simulink model "QUAD_With_MPC_Final"  (R2015a)
settings: Solver=ode45  StartTime=0.0  StopTime=120  RelTol=1e-3
libraries: simulink x6, commnoisgen2 x5, mpclib x1
settings Model: SimulationMode=accelerator  Creator=Oussama  LastModifiedBy=Oussama

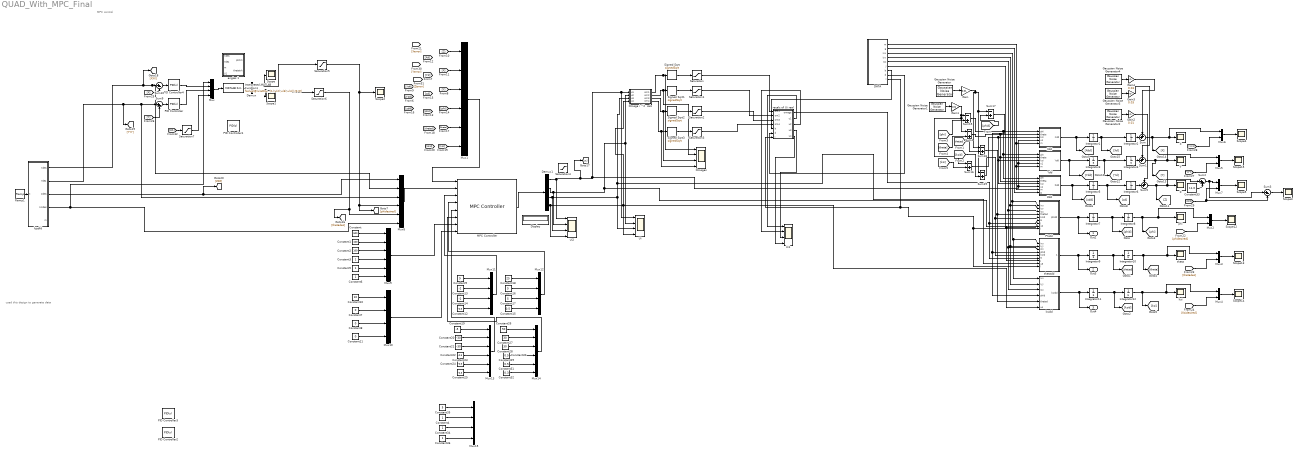
== system QUAD_With_MPC_Final ==
  note: MPC control
  note: used this design to generate data
  Constant : Constant  Value=500
  Constant1 : Constant  Value=100
  Constant10 : Constant  Value=10
  Constant11 : Constant  Value=0
  Constant12 : Constant  Value=-0.5
  Constant13 : Constant  Value=-2
  Constant14 : Constant  Value=-2
  Constant15 : Constant  Value=0.5
  Constant16 : Constant  Value=5
  Constant17 : Constant  Value=5
  Constant18 : Constant  Value=25
  Constant19 : Constant  Value=-5
  Constant2 : Constant  Value=100
  Constant20 : Constant  Value=-30
  Constant21 : Constant  Value=-30
  Constant{3..6,22,29,34,36} (8 alike) : Constant
  Constant23 : Constant  Value=-0.5
  Constant24 : Constant  Value=-0.5
  Constant25 : Constant  Value=-0.3
  Constant26 : Constant  Value=50
  Constant27 : Constant  Value=30
  Constant28 : Constant  Value=30
  Constant30 : Constant  Value=0.5
  Constant31 : Constant  Value=0.5
  Constant32 : Constant  Value=0.3
  Constant33 : Constant  Value=11.0
  Constant35 : Constant  Value=5
  Constant7 : Constant  Value=0
  Constant8 : Constant  Value=0
  Constant9 : Constant  Value=9
  DATA : MATLAB Function  TreatAsAtomicUnit=on
  Demux : Demux  Outputs=2
  Demux1 : Demux
  Display : Display
  Gain : Gain  Gain=0.01
  Gain1 : Gain  Gain=0.01
  Gain2 : Gain  Gain=0.01
  Gain3 : Gain  Gain=0.03
  Gain4 : Gain  Gain=0.03
  Gaussian Noise Generator : commnoisgen2/Gaussian Noise Generator  m=0  d=1  s=41  Ts=0.07  frameBased=off  sampPerFrame=1  orient=off  outDataType=double
  Gaussian Noise Generator1 : commnoisgen2/Gaussian Noise Generator  m=0  d=1  s=41  Ts=0.07  frameBased=off  sampPerFrame=1  orient=off  outDataType=double
  Gaussian Noise Generator2 : commnoisgen2/Gaussian Noise Generator  m=0.3  d=1  s=41  Ts=0.5  frameBased=off  sampPerFrame=1  orient=off  outDataType=double
  Gaussian Noise Generator3 : commnoisgen2/Gaussian Noise Generator  m=0.3  d=1  s=41  Ts=1.2  frameBased=off  sampPerFrame=1  orient=off  outDataType=double
  Gaussian Noise Generator4 : commnoisgen2/Gaussian Noise Generator  m=0.3  d=1  s=41  Ts=1  frameBased=off  sampPerFrame=1  orient=off  outDataType=double
  Integrator{1..12} (12 alike) : Integrator
  Interpreted MATLAB Function1 : MATLABFcn  MATLABFcn=fsolve(@(x)attitudes3(x,u(1),u(2),u(3),u(4)),[0,0])  OutputDimensions=2
  MPC Controller : mpclib/MPC Controller  SCDEnableBlockLinearizationSpecification=on  mpcobj=MPC2  is_multiple=0  enable_value=0  n_mv=4  n_mo=6  n_md=0  n_ts=0.02  is_designfromscratch=0  return_u0=off  ref_from_ws=off  ref_signal_name=[]  ref_preview=off  md_from_ws=off  md_signal_name=[]  md_preview=off  from_project=off  project_file=MPCtask.mat  md_inport=off  mv_inport=off  cost_outport=off  return_sequence=off  return_qpstatus=off  return_state=off  state_inport=off  lims_inport=on  ywt_inport=on  uwt_inport=off  duwt_inport=off  rhoeps_inport=off  uref_inport=on  BlockDataType=double  SampleTimeInherited=off  switch_inport=off
  Mux{,10..12,15} (5 alike) : Mux
  Mux{1,8..9,13..14} (5 alike) : Mux  Inputs=6
  Mux{2..7} (6 alike) : Mux  Inputs=2
  Omega i ^2  calc : MATLAB Function  TreatAsAtomicUnit=on
  Omegas : Scope  NumInputPorts=4
      settings: YMin=-5~-5~-5~-5  YMax=5~5~5~5  SaveName=ScopeData3
  PID Controller : simulink/Continuous/PID Controller  Controller=PID  TimeDomain=Continuous-time  SampleTime=-1  IntegratorMethod=Forward Euler  FilterMethod=Forward Euler  Form=Parallel  UseFilter=on  ControllerParametersSource=internal  P=0.7  I=0.4  D=1.8  N=100  InitialConditionSource=internal  InitialConditionForIntegrator=0  InitialConditionForFilter=0  ExternalReset=none  LimitOutput=off  UpperSaturationLimit=inf  LowerSaturationLimit=-inf  LinearizeAsGain=on  AntiWindupMode=none  Kb=1  TrackingMode=off  Kt=1  PParamMin=[]  PParamMax=[]  IParamMin=[]  IParamMax=[]  DParamMin=[]  DParamMax=[]  NParamMin=[]  NParamMax=[]  KbParamMin=[]  KbParamMax=[]  KtParamMin=[]  KtParamMax=[]  POutMin=[]  POutMax=[]  IOutMin=[]  IOutMax=[]  DOutMin=[]  DOutMax=[]  NOutMin=[]  NOutMax=[]  KbOutMin=[]  KbOutMax=[]  KtOutMin=[]  KtOutMax=[]  IntegratorOutMin=[]  IntegratorOutMax=[]  FilterOutMin=[]  FilterOutMax=[]  SumOutMin=[]  SumOutMax=[]  SumI1OutMin=[]  SumI1OutMax=[]  SumI2OutMin=[]  SumI2OutMax=[]  SumI3OutMin=[]  SumI3OutMax=[]  SumDOutMin=[]  SumDOutMax=[]  SaturationOutMin=[]  SaturationOutMax=[]  IntegratorContinuousStateAttributes=''  IntegratorStateMustResolveToSignalObject=off  IntegratorRTWStateStorageClass=Auto  FilterContinuousStateAttributes=''  FilterStateMustResolveToSignalObject=off  FilterRTWStateStorageClass=Auto  DifferentiatorICPrevScaledInput=0  DifferentiatorOutMin=[]  DifferentiatorOutMax=[]
  PID Controller1 : simulink/Continuous/PID Controller  Controller=PID  TimeDomain=Continuous-time  SampleTime=-1  IntegratorMethod=Forward Euler  FilterMethod=Forward Euler  Form=Parallel  UseFilter=on  ControllerParametersSource=internal  P=1  I=0.7  D=2.9  N=100  InitialConditionSource=internal  InitialConditionForIntegrator=0  InitialConditionForFilter=0  ExternalReset=none  LimitOutput=off  UpperSaturationLimit=inf  LowerSaturationLimit=-inf  LinearizeAsGain=on  AntiWindupMode=none  Kb=1  TrackingMode=off  Kt=1  PParamMin=[]  PParamMax=[]  IParamMin=[]  IParamMax=[]  DParamMin=[]  DParamMax=[]  NParamMin=[]  NParamMax=[]  KbParamMin=[]  KbParamMax=[]  KtParamMin=[]  KtParamMax=[]  POutMin=[]  POutMax=[]  IOutMin=[]  IOutMax=[]  DOutMin=[]  DOutMax=[]  NOutMin=[]  NOutMax=[]  KbOutMin=[]  KbOutMax=[]  KtOutMin=[]  KtOutMax=[]  IntegratorOutMin=[]  IntegratorOutMax=[]  FilterOutMin=[]  FilterOutMax=[]  SumOutMin=[]  SumOutMax=[]  SumI1OutMin=[]  SumI1OutMax=[]  SumI2OutMin=[]  SumI2OutMax=[]  SumI3OutMin=[]  SumI3OutMax=[]  SumDOutMin=[]  SumDOutMax=[]  SaturationOutMin=[]  SaturationOutMax=[]  IntegratorContinuousStateAttributes=''  IntegratorStateMustResolveToSignalObject=off  IntegratorRTWStateStorageClass=Auto  FilterContinuousStateAttributes=''  FilterStateMustResolveToSignalObject=off  FilterRTWStateStorageClass=Auto  DifferentiatorICPrevScaledInput=0  DifferentiatorOutMin=[]  DifferentiatorOutMax=[]
  PID Controller2 : simulink/Continuous/PID Controller  Controller=PID  TimeDomain=Continuous-time  SampleTime=-1  IntegratorMethod=Forward Euler  FilterMethod=Forward Euler  Form=Parallel  UseFilter=on  ControllerParametersSource=internal  P=0.5  I=0.1  D=0.25  N=100  InitialConditionSource=internal  InitialConditionForIntegrator=0  InitialConditionForFilter=0  ExternalReset=none  LimitOutput=off  UpperSaturationLimit=inf  LowerSaturationLimit=-inf  LinearizeAsGain=on  AntiWindupMode=none  Kb=1  TrackingMode=off  Kt=1  PParamMin=[]  PParamMax=[]  IParamMin=[]  IParamMax=[]  DParamMin=[]  DParamMax=[]  NParamMin=[]  NParamMax=[]  KbParamMin=[]  KbParamMax=[]  KtParamMin=[]  KtParamMax=[]  POutMin=[]  POutMax=[]  IOutMin=[]  IOutMax=[]  DOutMin=[]  DOutMax=[]  NOutMin=[]  NOutMax=[]  KbOutMin=[]  KbOutMax=[]  KtOutMin=[]  KtOutMax=[]  IntegratorOutMin=[]  IntegratorOutMax=[]  FilterOutMin=[]  FilterOutMax=[]  SumOutMin=[]  SumOutMax=[]  SumI1OutMin=[]  SumI1OutMax=[]  SumI2OutMin=[]  SumI2OutMax=[]  SumI3OutMin=[]  SumI3OutMax=[]  SumDOutMin=[]  SumDOutMax=[]  SaturationOutMin=[]  SaturationOutMax=[]  IntegratorContinuousStateAttributes=''  IntegratorStateMustResolveToSignalObject=off  IntegratorRTWStateStorageClass=Auto  FilterContinuousStateAttributes=''  FilterStateMustResolveToSignalObject=off  FilterRTWStateStorageClass=Auto  DifferentiatorICPrevScaledInput=0  DifferentiatorOutMin=[]  DifferentiatorOutMax=[]
  PID Controller3 : simulink/Continuous/PID Controller  Controller=PID  TimeDomain=Continuous-time  SampleTime=-1  IntegratorMethod=Forward Euler  FilterMethod=Forward Euler  Form=Parallel  UseFilter=on  ControllerParametersSource=internal  P=0.5  I=0.1  D=0.3  N=100  InitialConditionSource=internal  InitialConditionForIntegrator=0  InitialConditionForFilter=0  ExternalReset=none  LimitOutput=off  UpperSaturationLimit=inf  LowerSaturationLimit=-inf  LinearizeAsGain=on  AntiWindupMode=none  Kb=1  TrackingMode=off  Kt=1  PParamMin=[]  PParamMax=[]  IParamMin=[]  IParamMax=[]  DParamMin=[]  DParamMax=[]  NParamMin=[]  NParamMax=[]  KbParamMin=[]  KbParamMax=[]  KtParamMin=[]  KtParamMax=[]  POutMin=[]  POutMax=[]  IOutMin=[]  IOutMax=[]  DOutMin=[]  DOutMax=[]  NOutMin=[]  NOutMax=[]  KbOutMin=[]  KbOutMax=[]  KtOutMin=[]  KtOutMax=[]  IntegratorOutMin=[]  IntegratorOutMax=[]  FilterOutMin=[]  FilterOutMax=[]  SumOutMin=[]  SumOutMax=[]  SumI1OutMin=[]  SumI1OutMax=[]  SumI2OutMin=[]  SumI2OutMax=[]  SumI3OutMin=[]  SumI3OutMax=[]  SumDOutMin=[]  SumDOutMax=[]  SaturationOutMin=[]  SaturationOutMax=[]  IntegratorContinuousStateAttributes=''  IntegratorStateMustResolveToSignalObject=off  IntegratorRTWStateStorageClass=Auto  FilterContinuousStateAttributes=''  FilterStateMustResolveToSignalObject=off  FilterRTWStateStorageClass=Auto  DifferentiatorICPrevScaledInput=0  DifferentiatorOutMin=[]  DifferentiatorOutMax=[]
  PID Controller4 : simulink/Continuous/PID Controller  Controller=PID  TimeDomain=Continuous-time  SampleTime=-1  IntegratorMethod=Forward Euler  FilterMethod=Forward Euler  Form=Parallel  UseFilter=on  ControllerParametersSource=internal  P=0.7  I=0.4  D=1.8  N=100  InitialConditionSource=internal  InitialConditionForIntegrator=0  InitialConditionForFilter=0  ExternalReset=none  LimitOutput=off  UpperSaturationLimit=inf  LowerSaturationLimit=-inf  LinearizeAsGain=on  AntiWindupMode=none  Kb=1  TrackingMode=off  Kt=1  PParamMin=[]  PParamMax=[]  IParamMin=[]  IParamMax=[]  DParamMin=[]  DParamMax=[]  NParamMin=[]  NParamMax=[]  KbParamMin=[]  KbParamMax=[]  KtParamMin=[]  KtParamMax=[]  POutMin=[]  POutMax=[]  IOutMin=[]  IOutMax=[]  DOutMin=[]  DOutMax=[]  NOutMin=[]  NOutMax=[]  KbOutMin=[]  KbOutMax=[]  KtOutMin=[]  KtOutMax=[]  IntegratorOutMin=[]  IntegratorOutMax=[]  FilterOutMin=[]  FilterOutMax=[]  SumOutMin=[]  SumOutMax=[]  SumI1OutMin=[]  SumI1OutMax=[]  SumI2OutMin=[]  SumI2OutMax=[]  SumI3OutMin=[]  SumI3OutMax=[]  SumDOutMin=[]  SumDOutMax=[]  SaturationOutMin=[]  SaturationOutMax=[]  IntegratorContinuousStateAttributes=''  IntegratorStateMustResolveToSignalObject=off  IntegratorRTWStateStorageClass=Auto  FilterContinuousStateAttributes=''  FilterStateMustResolveToSignalObject=off  FilterRTWStateStorageClass=Auto  DifferentiatorICPrevScaledInput=0  DifferentiatorOutMin=[]  DifferentiatorOutMax=[]
  Phidd : MATLAB Function  TreatAsAtomicUnit=on
  Ramp1 : simulink/Sources/Ramp  slope=1  start=0  X0=0
  Saturation{,1..3} (4 alike) : Saturate  UpperLimit=5000  LowerLimit=0
  Saturation4 : Saturate  UpperLimit=50  LowerLimit=5
  Saturation5 : Saturate  UpperLimit=0.4  LowerLimit=-0.4
  Saturation6 : Saturate
  Saturation7 : Saturate  UpperLimit=50  LowerLimit=0.5
  Scope{,1..5,12..15} (10 alike) : Scope
      Scope settings: TimeRange=10  YMin=-0.504  YMax=-0.491
      Scope1 settings: YMin=1.49226  YMax=1.64934
      Scope12 settings: YMin=-0.00625  YMax=-0.00425  SaveName=phi_ang
      Scope13 settings: YMin=-0.07  YMax=0.05  SaveName=theta_ang
      Scope14 settings: YMin=0  YMax=7e-13  SaveName=psi_ang
      Scope15 settings: YMin=-9.78  YMax=-9.65  SaveName=ydata
      Scope2 settings: YMin=1.49226  YMax=1.64934  SaveName=ScopeData8
      Scope3 settings: YMin=-12.016  YMax=-12.006  SaveName=zdata1
      Scope4 settings: TimeRange=44.14385330578512  YMin=0  YMax=13  SaveName=xdata
      Scope5 settings: YMin=7.95  YMax=8.5  SaveName=zdata
  Signed Sqrt{,1..3} (4 alike) : Sqrt  Operator=signedSqrt  SaturateOnIntegerOverflow=on
  Sum : Sum  Inputs=++|
  Sum1 : Sum  Inputs=++|
  Sum10 : Sum  Inputs=|+-
  Sum{4,15..19} (6 alike) : Sum  Inputs=-+
  Sum2 : Sum  Inputs=|++
  Sum3 : Sum  Inputs=|+-
  Sum5 : Sum  Inputs=++|
  Sum9 : Sum  Inputs=|+-
  Ui : Scope  NumInputPorts=4
      settings: YMin=-5~-5~-5~-5  YMax=5~5~5~5  SaveName=ScopeData15
  Ui1 : Scope  NumInputPorts=4
      settings: YMin=-5~-5~-5~-5  YMax=5~5~5~5  SaveName=ScopeData4
  Ui2 : Scope  NumInputPorts=4
      settings: YMin=-5~-5~-5~-5  YMax=5~5~5~5  SaveName=ScopeData7
  X : Scope
      settings: YMin=3.81  YMax=3.95  SaveName=ScopeData6
  Xdd : MATLAB Function  TreatAsAtomicUnit=on
  Y : Scope
      settings: YMin=-0.01095  YMax=-0.0103  SaveName=ScopeData5
  Ydd : MATLAB Function  TreatAsAtomicUnit=on
  "Z " : Scope
      settings: YMin=7.615  YMax=7.6215  SaveName=ScopeData2
  Zdd : MATLAB Function  TreatAsAtomicUnit=on
  angles 1 : MATLAB Function  TreatAsAtomicUnit=on
  "hjsdfd " : MATLAB Function  TreatAsAtomicUnit=on
  ksi : Scope
      settings: SaveName=ksiangle
  ksidd : MATLAB Function  TreatAsAtomicUnit=on
  phi : Scope
      settings: SaveName=phiangle
  recalc of Ui real : MATLAB Function  TreatAsAtomicUnit=on
  theta : Scope
      settings: SaveName=thetaangle
  thetadd : MATLAB Function  TreatAsAtomicUnit=on
  Out2 : Outport
  Out3 : Outport  Port=2
  Out4 : Outport  Port=3
  wires:
  Saturation/1 -> recalc of Ui real/1(om1)
  Saturation1/1 -> recalc of Ui real/2(om2)
  Saturation2/1 -> recalc of Ui real/3(om3)
  Signed Sqrt/1 -> Saturation/1
  Signed Sqrt1/1 -> Saturation1/1
  Signed Sqrt2/1 -> Saturation2/1
  Signed Sqrt3/1 -> Saturation3/1
  Xdd/1(Xdd) -> [Xdd], Integrator1/1
  Ydd/1(Ydd) -> [Ydd], Integrator3/1
  Zdd/1(Zdd) -> [zdd], Integrator5/1
  Phidd/1(phidd) -> Out2/1, Integrator7/1
  Integrator7/1 -> [phid], Integrator8/1
  thetadd/1(thetadd) -> Out3/1, Integrator9/1
  Integrator9/1 -> [thetad], Integrator10/1
  ksidd/1(ksidd) -> Out4/1, Integrator11/1
  Integrator11/1 -> [ksid], Integrator12/1
  Integrator8/1 -> Mux2/1, phi/1, [phi]
  DATA/1(m) -> Zdd/5(m), Ydd/5(m), Xdd/5(m)
  DATA/2(g) -> Zdd/6(g)
  DATA/3(Ixx) -> ksidd/1(Ixx), thetadd/1(Ixx), Phidd/1(Ixx)
  DATA/4(Iyy) -> Phidd/2(Iyy), ksidd/2(Iyy), thetadd/2(Iyy)
  DATA/5(Izz) -> thetadd/3(Izz), ksidd/3(Izz), Phidd/3(Izz)
  DATA/6(J) -> thetadd/7(J), Phidd/7(J)
  Sum15/1 -> Zdd/1(phi), Ydd/1(phi), Xdd/1(phi)
  Sum4/1 -> Zdd/2(theta), Ydd/2(theta), Xdd/2(theta)
  Sum16/1 -> Ydd/3(ksi), Zdd/3(ksi), Xdd/3(ksi)
  Sum18/1 -> Phidd/4(thetad), ksidd/5(thetad)
  Sum19/1 -> Phidd/5(ksid), thetadd/5(ksid)
  Sum17/1 -> ksidd/4(phid), thetadd/4(phid)
  recalc of Ui real/1(omega) -> thetadd/6(omega), Phidd/6(omega)
  DATA/7(b) -> recalc of Ui real/5(b)
  DATA/8(d) -> recalc of Ui real/6(d)
  Demux1/4 -> Ui2/4, Omega i ^2  calc/4(u4), Ui/4, ksidd/6(u4)
  Demux1/3 -> Ui2/3, Omega i ^2  calc/3(u3), thetadd/8(u3), Ui/3
  Demux1/2 -> Ui2/2, Phidd/8(u2), Omega i ^2  calc/2(u2), Ui/2
  Omega i ^2  calc/1(om1) -> Omegas/1, Signed Sqrt/1
  Omega i ^2  calc/2(om2) -> Omegas/2, Signed Sqrt1/1
  Omega i ^2  calc/3(om3) -> Omegas/3, Signed Sqrt2/1
  Omega i ^2  calc/4(om4) -> Omegas/4, Signed Sqrt3/1
  Gain1/1 -> Sum16/1, Sum4/1, Sum15/1
  [phi] -> Sum15/2
  [theta] -> Sum4/2
  [ksi] -> Sum16/2
  Gain/1 -> Sum19/1, Sum17/1, Sum18/1
  [phid] -> Sum17/2
  [thetad] -> Sum18/2
  [ksid] -> Sum19/2
  Integrator5/1 -> [zd], Integrator6/1
  Integrator3/1 -> [Yd], Integrator4/1
  Integrator1/1 -> [Xd], Integrator2/1
  DATA/9(l) -> Phidd/9(l), thetadd/9(l), recalc of Ui real/7(l)
  [phidesired] -> Mux2/2
  Mux2/1 -> Scope12/1
  Integrator10/1 -> [theta], Mux3/1, theta/1
  [thetades] -> Mux3/2
  Mux3/1 -> Scope13/1
  Integrator12/1 -> [ksi], Mux4/1, ksi/1
  [Ksidesired] -> Mux4/2
  Mux4/1 -> Scope14/1
  "hjsdfd "/1(Xdes) -> Mux8/2, Sum10/1, [XXX]
  [X] -> Sum10/2
  "hjsdfd "/2(Ydes) -> Mux8/3, Sum9/1, [YYY]
  [Y] -> Sum9/2
  Mux5/1 -> Scope15/1
  Sum/1 -> [X], Mux6/1, X/1
  [XXX] -> Mux6/2
  [ZZZ] -> Sum3/2, Mux7/2
  [X] -> Mux1/2
  [Y] -> Mux1/3
  [phi] -> Mux1/4
  [theta] -> Mux1/5
  [ksi] -> Mux1/6
  Mux1/1 -> MPC Controller/1
  Mux8/1 -> MPC Controller/2
  MPC Controller/1 -> Demux1/1
  Mux/1 -> Interpreted MATLAB Function1/1
  Demux/1 -> Scope/1, Saturation5/1
  Demux/2 -> Saturation6/1, Scope1/1
  Interpreted MATLAB Function1/1 -> Demux/1
  "hjsdfd "/4(ksides) -> Mux/1, Mux8/6
  Sum10/1 -> PID Controller4/1
  Sum9/1 -> PID Controller/1
  Saturation6/1 -> Mux8/5, [thetades]
  Saturation5/1 -> Scope2/1, Mux8/4, [phidesired]
  Sum1/1 -> [Y], Mux5/1, Y/1
  [YYY] -> Mux5/2
  Sum5/1 -> [Z], Sum2/1, "Z "/1
  Mux7/1 -> Scope5/1
  Saturation3/1 -> recalc of Ui real/4(om4)
  Mux9/1 -> MPC Controller/7
  Constant/1 -> Mux9/1
  Constant1/1 -> Mux9/2
  Constant2/1 -> Mux9/3
  Constant3/1 -> Mux9/4
  Constant5/1 -> Mux9/5
  Constant6/1 -> Mux9/6
  Mux10/1 -> MPC Controller/8
  Constant7/1 -> Mux10/2
  Constant8/1 -> Mux10/3
  Constant10/1 -> Mux10/1
  Constant11/1 -> Mux10/4
  Mux11/1 -> MPC Controller/3
  Constant13/1 -> Mux11/2
  Constant14/1 -> Mux11/3
  Constant9/1 -> Mux11/1
  Constant12/1 -> Mux11/4
  Constant16/1 -> Mux12/2
  Constant17/1 -> Mux12/3
  Constant18/1 -> Mux12/1
  Constant15/1 -> Mux12/4
  Mux12/1 -> MPC Controller/4
  Mux13/1 -> MPC Controller/5
  Constant19/1 -> Mux13/1
  Constant20/1 -> Mux13/2
  Constant21/1 -> Mux13/3
  Constant22/1 -> Mux13/4
  Constant24/1 -> Mux13/5
  Constant25/1 -> Mux13/6
  Mux14/1 -> MPC Controller/6
  Constant26/1 -> Mux14/1
  Constant27/1 -> Mux14/2
  Constant28/1 -> Mux14/3
  Constant29/1 -> Mux14/4
  Constant31/1 -> Mux14/5
  Constant32/1 -> Mux14/6
  recalc of Ui real/2(u1) -> Ui1/1
  recalc of Ui real/3(u2) -> Ui1/2
  recalc of Ui real/4(u3) -> Ui1/3
  recalc of Ui real/5(u4) -> Ui1/4
  PID Controller/1 -> Mux/3
  PID Controller4/1 -> Mux/2
  "hjsdfd "/3(Zdes) -> [ZZZ], Mux8/1
  Sum2/1 -> Sum3/1, Mux7/1
  Constant33/1 -> Sum2/2
  Sum3/1 -> Scope3/1
  [Z] -> Mux1/1
  Constant4/1 -> Mux15/2
  Constant34/1 -> Mux15/3
  Constant35/1 -> Mux15/1
  Constant36/1 -> Mux15/4
  [U1] -> Saturation7/1
  Saturation7/1 -> Mux/4
  Mux6/1 -> Scope4/1
  Ramp1/1 -> "hjsdfd "/1(t)
  Gaussian Noise Generator2/1 -> Gain2/1
  Gain2/1 -> Sum5/1
  Gaussian Noise Generator3/1 -> Gain3/1
  Gain3/1 -> Sum1/1
  Gaussian Noise Generator4/1 -> Gain4/1
  Gain4/1 -> Sum/1
  Gaussian Noise Generator/1 -> Gain/1
  Gaussian Noise Generator1/1 -> Gain1/1
  Integrator2/1 -> Sum/2
  Integrator4/1 -> Sum1/2
  Integrator6/1 -> Sum5/2
  Demux1/1 -> [U1], Zdd/4(u1), Ydd/4(u1), Xdd/4(u1), Omega i ^2  calc/1(u1), Ui/1, Ui2/1

== matlab function QUAD_With_MPC_Final/Ydd ==
  data: phi input; Ydd output; theta input; ksi input; u1 input; m input
function Ydd = fcn(phi,theta, ksi,u1,m)
m=1;

Ydd=(-cos(ksi)*sin(phi)+sin(ksi)*sin(theta)*cos(phi))*u1/m;

== matlab function QUAD_With_MPC_Final/Zdd ==
  data: phi input; Zdd output; theta input; ksi input; u1 input; m input; g input
function Zdd = fcn(phi,theta, ksi,u1,m,g)
m=1;
g=9.81;

Zdd=-g+(cos(theta)*cos(phi))*u1/m;

== matlab function QUAD_With_MPC_Final/DATA ==
  data: m output; g output; Ixx output; Iyy output; Izz output; J output; b output; d output; l output
function [m,g,Ixx,Iyy,Izz,J,b,d,l] = fcn
m=1;
g=9.81;

Ixx=1*0.008;
Iyy=1*0.008;
Izz=1*0.015;
b=0.0001;
d=0.000001;
l=0.25;
J=0.0001;

== matlab function QUAD_With_MPC_Final/Phidd ==
  data: Ixx input; Iyy input; phidd output; Izz input; thetad input; ksid input; omega input; J input; u2 input; l input
function phidd = fcn(Ixx,Iyy,Izz,thetad, ksid,omega,J,u2,l)


phidd=1/Ixx*((Iyy-Izz)*thetad*ksid-J*thetad*omega+l*u2);

== matlab function QUAD_With_MPC_Final/thetadd ==
  data: Ixx input; Iyy input; thetadd output; Izz input; phid input; ksid input; omega input; J input; u3 input; l input
function thetadd = fcn(Ixx,Iyy,Izz,phid, ksid,omega,J,u3,l)


thetadd=1/Iyy*((Izz-Ixx)*phid*ksid+J*phid*omega+l*u3);

== matlab function QUAD_With_MPC_Final/ksidd ==
  data: Ixx input; Iyy input; ksidd output; Izz input; phid input; thetad input; u4 input
function ksidd = fcn(Ixx,Iyy,Izz,phid, thetad,u4)


ksidd=1/Izz*((Ixx-Iyy)*phid*thetad+u4);

== matlab function QUAD_With_MPC_Final/Omega i ^2  calc ==
  data: u1 input; om1 output; u2 input; u3 input; u4 input; om2 output; om3 output; om4 output
function [om1,om2,om3,om4] = fcn(u1,u2,u3,u4)
%#codegen
b=0.0001;
d=0.000001;
l=0.25;
A=[ 1/(4*b),0, -1/(2*b*l), -1/(4*d);1/(4*b), -1/(2*b*l),0,  1/(4*d); 1/(4*b),  0,  1/(2*b*l), -1/(4*d);1/(4*b),1/(2*b*l), 0,  1/(4*d)];
B=A*[u1;u2;u3;u4];
%[om1;om2;om3;om4]
om1= B(1);
om2=B(2);
om3=B(3);
om4=B(4);

== matlab function QUAD_With_MPC_Final/Xdd ==
  data: phi input; Xdd output; theta input; ksi input; u1 input; m input
function Xdd = fcn(phi,theta, ksi,u1,m)


Xdd=(sin(ksi)*sin(phi)+cos(ksi)*sin(theta)*cos(phi))*u1/m;

== matlab function QUAD_With_MPC_Final/recalc of Ui real ==
  data: om1 input; omega output; om2 input; om3 input; om4 input; b input; d input; l input; u1 output; u2 output; u3 output; u4 output
function [omega, u1,u2,u3,u4] = fcn(om1,om2,om3,om4,b,d,l)


omega=-om1+om2-om3+om4;
u1=b*(om1^2+om2^2+om3^2+om4^2);
u2=l*b*(om4^2-om2^2);
u3=l*b*(om3^2-om1^2);
u4=d*(om4^2+om2^2-om1^2-om3^2);

== matlab function QUAD_With_MPC_Final/hjsdfd  ==
  data: t input; Xdes output; Ydes output; Zdes output; ksides output; m output
function [Xdes,Ydes,Zdes,ksides,m] = fcn(t)

A=15;a=5;
B=10;b=4;
C=8;c=5;
fr=0.05;
Xdes=A*cos(a*fr*t);
Ydes=B*sin(b*fr*t);
Zdes=C*(1-exp(-5*fr*t));
%#codegen
m=1;
%ksides=0.2*cos(0.1*time)-0.32*sin(0.2*time);
ksides=0;
%plot3(Xdes,Ydes,Zdes,'*')
%hold on
%grid on

== matlab function QUAD_With_MPC_Final/angles 1 ==
  data: Xdes input; phitrk output; Ydes input; m input; U1 input; thetatrk output
function [phitrk,thetatrk]  = fcn(Xdes,Ydes, m,U1)
%#codegen
if U1<=5
    phitrk=0;
else
    if (abs(Ydes*m/U1) >= 0.3)
        phitrk= -sign(Ydes*m/U1)*pi/10;
    else
    phitrk=-asin(Ydes*m/U1);
    end
end
%%%%%%%%%%%%%%%%%%
if U1<=5
    thetatrk=0;
elseif (abs( Xdes*m/(U1*cos(phitrk)) ) >= 0.3 )
        thetatrk = sign( Xdes*m/(U1*cos(phitrk)) )*pi/10 ;
    else
    thetatrk=asin(Xdes*m/(U1*cos(phitrk)) );
end

    
%%%%%%%%%%%%
if phitrk > pi/3
    phitrk=pi/3;
end
if phitrk < -pi/3
    phitrk=-pi/3;
end
%%%%%%%%%%%%%%%
if thetatrk > pi/3
    thetatrk=pi/3;
end
if thetatrk < -pi/3
    thetatrk=-pi/3;
end
